simulink model "final_simulink_model_V3"  (R2022a)
settings: Solver=FixedStepAuto  StartTime=0.0  StopTime=inf  FixedStep=0.001  RelTol=1e-3  EnableMultiTasking=on
values from neighbouring files (symbols this model uses):
  data = double(raw_data(1)/100)    [readBleDataCallback.m]
libraries: simulink x4, vrlib x2
settings Model: ExtModeTrigDuration=2  Creator=Jacopo  LastModifiedBy=Filippo
settings SolverCC: AlgebraicLoopSolver=TrustRegion  AutoInsertRateTranBlk=on
settings OptimizationCC: DefaultParameterBehavior=Inlined  EnhancedBackFolding=on  PassReuseOutputArgsThreshold=0  MaxStackSize=64  OptimizeBlockOrder=speed  DifferentSizesBufferReuse=on  OptimizationCustomize=off
settings DebuggingCC: ParameterTunabilityLossMsg=error  UnconnectedInputMsg=warning  UnconnectedOutputMsg=warning  UnconnectedLineMsg=warning  SFMachineParentedDataDiag=warning
settings HardwareCC: ProdBitPerInt=16  ProdBitPerPointer=16  ProdBitPerSizeT=16  ProdBitPerPtrDiffT=16  ProdLargestAtomicFloat=None  ProdWordSize=8  ProdHWDeviceType=Atmel->AVR  UseEmbeddedCoderFeatures=off  UseSimulinkCoderFeatures=off
settings SFSimCC: MATLABDynamicMemAlloc=off
settings RTWCC: SystemTargetFile=ert.tlc  TemplateMakefile=ert_default_tmf  GenerateReport=on  Toolchain=Arduino AVR  BuildConfiguration=Faster Runs  LaunchReport=on
settings CodeAppCC: ForceParamTrailComments=on  OperatorAnnotations=on
settings ERTTargetCC: ERTCustomFileBanners=off  SupportContinuousTime=on  SupportNonInlinedSFcns=on  RemoveResetFunc=off  SupportVariableSizeSignals=on  ModelStepFunctionPrototypeControlCompliant=off  ExtModeStaticAllocSize=250  ERTCustomFileTemplate=example_file_process.tlc

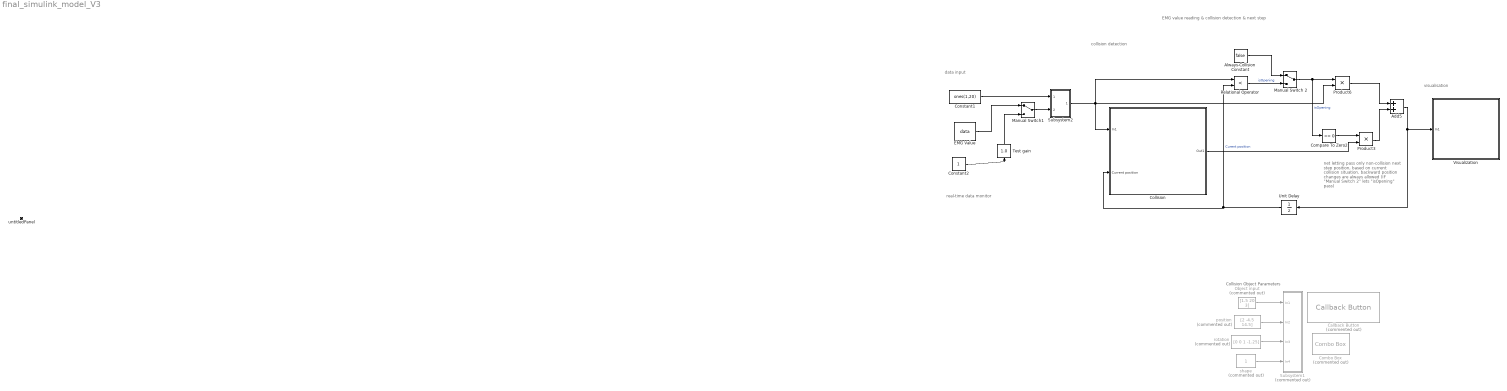
== system final_simulink_model_V3 ==
  note: real-time data monitor
  note: visualisation
  note: collision detection
  note: data input
  note: Collision Object Parameters
  note: EMG value reading & collision detection & next step
  note: net letting pass only non-collision next step position, based on current collision situation.
      | backward position changes are always allowed (IF "Manual Switch 2" lets "isOpening" pass)
  Add5 : Sum
  Always-Collision Constant : Constant  Value=false
  Callback Button : CallbackButton  Commented=on  ButtonText=Load Object
      settings: ClickFcn=|
      | inputParameters = str2num(get_param('final_simulink_model_V3/Object input', 'Value'));
      | position = str2num(get_param('final_simulink_model_V3/position', 'Value'));
      | rotation = str2num(get_param('final_simulink_model_V3/rotation', 'Value'));
      | shape = str2num(get_param('final_simulink_model_V3/shape', 'Value'));
      | 
      | changeCollisionObj_F(inputParameters, shape, position, rotation);
      | % set_param('final_simulink_model_V3/Subsystem/reload ball constant','Value','1');
      | set_param('final_simulink_model_V3/reload ball constant','Value','1');
  Collision : Subsystem  TreatAsAtomicUnit=on  SystemSampleTime=1
  Combo Box : ComboBox  Commented=on  SelectedLabel=Box
      settings: Values={{'Sphere', 'Box'}, [0 1]}
  Compare To Zero2 : simulink/Logic and Bit Operations/Compare To Zero  relop=<=  OutDataTypeStr=boolean
  Constant1 : Constant  Value=ones(1,20)
  Constant2 : Constant
  EMG Value : Constant  Value=data  OutMin=0  OutMax=1
  Manual Switch 2 : ManualSwitch
  Manual Switch1 : ManualSwitch
  Object input : Constant  Commented=on  Value=[1.5 20 3]  VectorParams1D=off  SampleTime=1
  Product3 : Product
  Product6 : Product
  Relational Operator : RelationalOperator  Operator=<  OutDataTypeStr=boolean  RndMeth=Simplest  InputSameDT=off
  Subsystem1 : Subsystem  Commented=on
  Subsystem2 : Subsystem  TreatAsAtomicUnit=on  SystemSampleTime=1
  Test gain : simulink/Math Operations/Slider Gain  gain=1.0  low=0  high=1
  Unit Delay : UnitDelay  InitialCondition=[0 0 0 0 0 0 0 0 0 0 0 0 0 0 0 0 0 0 0 0]'  SampleTime=-1  HasFrameUpgradeWarning=on
  Visualization : Subsystem  TreatAsAtomicUnit=on  SystemSampleTime=3
  position : Constant  Commented=on  Value=[2 -4.5 14.5]  SampleTime=1
  rotation : Constant  Commented=on  Value=[0 0 1 -1.25]  SampleTime=1
  shape : Constant  Commented=on  SampleTime=1
  untitledPanel : Subsystem  Tag=HiddenForWebPanel  IsWebBlockPanel=on
  wires:
  Object input/1 -> Subsystem1/1(In1)
  position/1 -> Subsystem1/2(In2)
  rotation/1 -> Subsystem1/3(In3)
  shape/1 -> Subsystem1/4(In4)
  Add5/1 -> Unit Delay/1, Visualization/1(In1)
  Constant1/1 -> Subsystem2/1(In1)
  Collision/1(Out1) -> Product3/2
  Compare To Zero2/1 -> Product3/1
  Product6/1 -> Add5/1
  Subsystem2/1(Out1) -> Collision/1(In1), Product6/2, Relational Operator/1
  Product3/1 -> Add5/2
  Manual Switch 2/1 -> Compare To Zero2/1, Product6/1  "isOpening"
  Unit Delay/1 -> Relational Operator/2, Collision/2(Current position)  "Curent position"
  EMG Value/1 -> Manual Switch1/1
  Relational Operator/1 -> Manual Switch 2/2  "isOpening"
  Always-Collision Constant/1 -> Manual Switch 2/1
  Constant2/1 -> Test gain/1
  Manual Switch1/1 -> Subsystem2/2(In2)
  Test gain/1 -> Manual Switch1/2

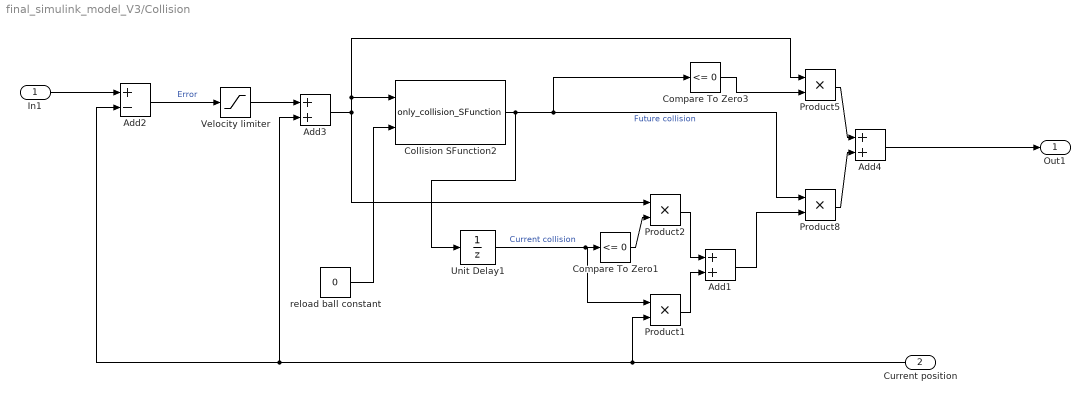
== system final_simulink_model_V3/Collision ==
  In1 : Inport
  Current position : Inport  Port=2
  Add1 : Sum
  Add2 : Sum  Inputs=+-
  Add3 : Sum
  Add4 : Sum
  Collision SFunction2 : M-S-Function  FunctionName=only_collision_SFunction
  Compare To Zero1 : simulink/Logic and Bit Operations/Compare To Zero  relop=<=  OutDataTypeStr=boolean
  Compare To Zero3 : simulink/Logic and Bit Operations/Compare To Zero  relop=<=  OutDataTypeStr=boolean
  Product1 : Product
  Product2 : Product
  Product5 : Product  OutDataTypeStr=double
  Product8 : Product
  Unit Delay1 : UnitDelay  InitialCondition=[0 0 0 0 0 0 0 0 0 0 0 0 0 0 0 0 0 0 0 0]'  SampleTime=-1  HasFrameUpgradeWarning=on
  Velocity limiter : Saturate  UpperLimit="[0.2247 0.1098 0.3023 0.4*0.3023  0 0.352 0.3178 0.4*0.3178  0 0.4422 0.2971 0.4*0.2971 0 0.3792 0.2754 0.4*0.2754 0 0.3905 0.3292 0.4*0.3292]'*0.2"  LowerLimit="[0.2247 0.1098 0.3023 0.4*0.3023  0 0.352 0.3178 0.4*0.3178  0 0.4422 0.2971 0.4*0.2971 0 0.3792 0.2754 0.4*0.2754 0 0.3905 0.3292 0.4*0.3292]'*(-0.2)"
  reload ball constant : Constant  Value=0
  Out1 : Outport
  wires:
  Velocity limiter/1 -> Add3/1
  Product1/1 -> Add1/2
  Current position/1 -> Add2/2, Add3/2, Product1/2
  Collision SFunction2/1 -> Unit Delay1/1, Compare To Zero3/1, Product8/1  "Future collision"
  Compare To Zero3/1 -> Product5/2
  Product5/1 -> Add4/1
  Compare To Zero1/1 -> Product2/2
  reload ball constant/1 -> Collision SFunction2/2
  Add4/1 -> Out1/1
  Add2/1 -> Velocity limiter/1  "Error"
  Product2/1 -> Add1/1
  Add3/1 -> Collision SFunction2/1, Product5/1, Product2/1
  Unit Delay1/1 -> Product1/1, Compare To Zero1/1  "Current collision"
  Add1/1 -> Product8/2
  Product8/1 -> Add4/2
  In1/1 -> Add2/1

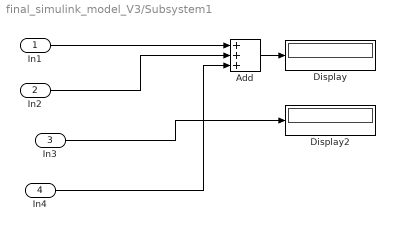
== system final_simulink_model_V3/Subsystem1 ==
  In1 : Inport
  In2 : Inport  Port=2
  In3 : Inport  Port=3
  In4 : Inport  Port=4
  Add : Sum  Inputs=+++
  Display : Display
  Display2 : Display
  wires:
  In4/1 -> Add/3
  Add/1 -> Display/1
  In2/1 -> Add/2
  In1/1 -> Add/1
  In3/1 -> Display2/1

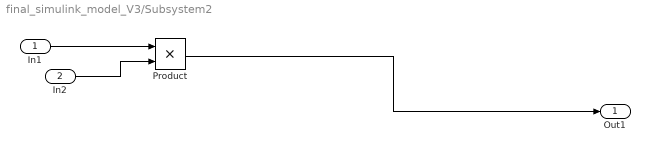
== system final_simulink_model_V3/Subsystem2 ==
  In1 : Inport
  In2 : Inport  Port=2
  Product : Product
  Out1 : Outport
  wires:
  In1/1 -> Product/1
  In2/1 -> Product/2
  Product/1 -> Out1/1

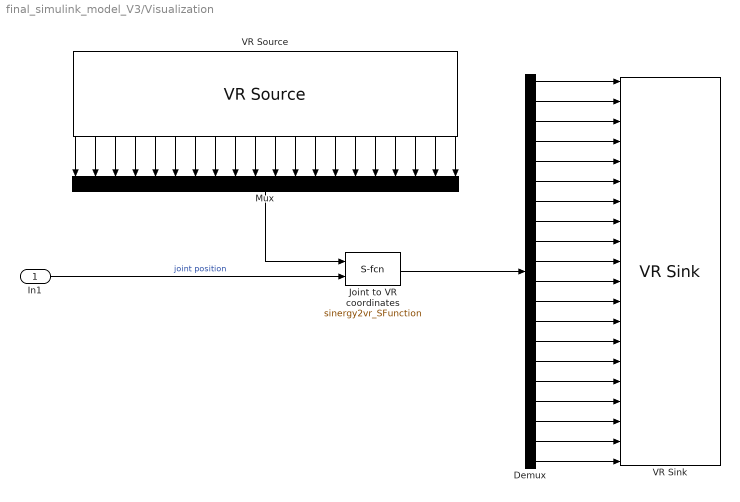
== system final_simulink_model_V3/Visualization ==
  In1 : Inport
  Demux : Demux  Outputs=20
  Joint to VR coordinates : M-S-Function  FunctionName=sinergy2vr_SFunction
  Mux : Mux  Inputs=20
  VR Sink : vrlib/VR Sink  InstantiateOnLoad=on  SampleTime=-1  ViewEnable=on  RemoteChange=off  RemoteView=off  FieldsWritten=body1.rotation.4.1.1.double#body2.rotation.4.1.1.double#body3.rotation.4.1.1.double#body4.rotation.4.1.1.double#body6.rotation.4.1.1.double#body7.rotation.4.1.1.double#body8.rotation.4.1.1.double#body9.rotation.4.1.1.double#body11.rotation.4.1.1.double#body12.rotation.4.1.1.double#body13.rotation.4.1.1.double#body14.rotation.4.1.1.double#body16.rotation.4.1.1.double#body17.rotation.4.1.1.double#body18.rotation.4.1.1.double#body19.rotation.4.1.1.double#body21.rotation.4.1.1.double#body22.rotation.4.1.1.double#body23.rotation.4.1.1.double#body24.rotation.4.1.1.double  WorldFileName=robot_sim.x3d  WorldDescription=Simple Robot Scene  AutoView=off  VideoDimensions=[]  AllowVariableSize=off
  VR Source : vrlib/VR Source  InstantiateOnLoad=on  SampleTime=-1  ViewEnable=on  RemoteChange=off  RemoteView=off  FieldsRead=body1.rotation.1.4.1.double#body2.rotation.1.4.1.double#body3.rotation.1.4.1.double#body4.rotation.1.4.1.double#body6.rotation.1.4.1.double#body7.rotation.1.4.1.double#body8.rotation.1.4.1.double#body9.rotation.1.4.1.double#body11.rotation.1.4.1.double#body12.rotation.1.4.1.double#body13.rotation.1.4.1.double#body14.rotation.1.4.1.double#body16.rotation.1.4.1.double#body17.rotation.1.4.1.double#body18.rotation.1.4.1.double#body19.rotation.1.4.1.double#body21.rotation.1.4.1.double#body22.rotation.1.4.1.double#body23.rotation.1.4.1.double#body24.rotation.1.4.1.double  WorldFileName=robot_sim.x3d  WorldDescription=Simple Robot Scene  AutoView=off  VideoDimensions=[]  AllowVariableSize=off
      settings: SourceProductBaseCode=SL
  wires:
  VR Source/15 -> Mux/15
  VR Source/8 -> Mux/8
  VR Source/4 -> Mux/4
  Mux/1 -> Joint to VR coordinates/1
  VR Source/20 -> Mux/20
  VR Source/16 -> Mux/16
  VR Source/2 -> Mux/2
  VR Source/11 -> Mux/11
  VR Source/19 -> Mux/19
  VR Source/6 -> Mux/6
  VR Source/17 -> Mux/17
  VR Source/14 -> Mux/14
  VR Source/12 -> Mux/12
  VR Source/5 -> Mux/5
  VR Source/13 -> Mux/13
  VR Source/7 -> Mux/7
  VR Source/9 -> Mux/9
  VR Source/10 -> Mux/10
  VR Source/3 -> Mux/3
  VR Source/1 -> Mux/1
  VR Source/18 -> Mux/18
  Joint to VR coordinates/1 -> Demux/1
  In1/1 -> Joint to VR coordinates/2  "joint position"
  Demux/12 -> VR Sink/12
  Demux/11 -> VR Sink/11
  Demux/13 -> VR Sink/13
  Demux/16 -> VR Sink/16
  Demux/19 -> VR Sink/19
  Demux/10 -> VR Sink/10
  Demux/8 -> VR Sink/8
  Demux/15 -> VR Sink/15
  Demux/1 -> VR Sink/1
  Demux/7 -> VR Sink/7
  Demux/20 -> VR Sink/20
  Demux/9 -> VR Sink/9
  Demux/6 -> VR Sink/6
  Demux/17 -> VR Sink/17
  Demux/5 -> VR Sink/5
  Demux/4 -> VR Sink/4
  Demux/18 -> VR Sink/18
  Demux/3 -> VR Sink/3
  Demux/14 -> VR Sink/14
  Demux/2 -> VR Sink/2

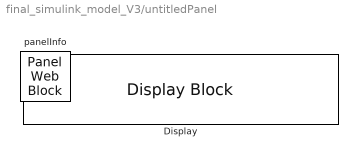
== system final_simulink_model_V3/untitledPanel ==
  Display : DisplayBlock  Tag=HiddenForWebPanel  PanelInfo="{\"panelId\":\"panelId-74e6be43-c473-4721-8b5b-9a4ba6cd94c4\",\"type\":\"panelChild\",\"version\":\"2019b\",\"zIndex\":1500002}"  LabelPosition=Hide  Transparency=1
  panelInfo : PanelWebBlock  Tag=HiddenForWebPanel  PanelInfo="{\"compacted\":false,\"height\":110,\"isActiveTab\":true,\"left\":25,\"name\":\"Panel\",\"panelId\":\"panelId-74e6be43-c473-4721-8b5b-9a4ba6cd94c4\",\"tabIndex\":0,\"tabbedSetId\":\"tabbedSet2731052545\",\"top\":550,\"type\":\"panel\",\"version\":\"2019b\",\"visible\":true,\"width\":355,\"zIndex\":1500002}"
